simulink model "Primerpunto_a"  (R2017b)
settings: Solver=VariableStepAuto  StartTime=0.0  StopTime=80  RelTol=1e-3
settings Model: Creator=HP  LastModifiedBy=franj
settings CodeAppCC: StateflowObjectComments=on

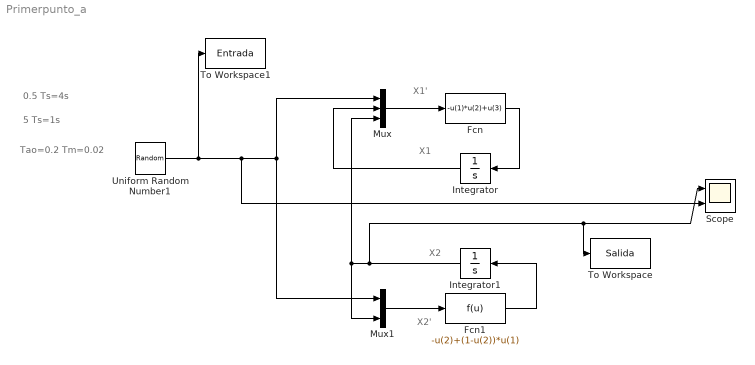
== system Primerpunto_a ==
  note: Tao=0.2
      | Tm=0.02
  note: 5 Ts=1s
  note: 0.5 Ts=4s
  note: X2'
  note: X2
  note: X1
  note: X1'
  Fcn : Fcn  Expr=-u(1)*u(2)+u(3)
  Fcn1 : Fcn  Expr=-u(2)+(1-u(2))*u(1)
  Integrator : Integrator
  Integrator1 : Integrator
  Mux : Mux  Inputs=3
  Mux1 : Mux  Inputs=2
  Scope : Scope  NumInputPorts=2
  To Workspace : ToWorkspace  VariableName=Salida  SampleTime=0.02
  To Workspace1 : ToWorkspace  VariableName=Entrada  SampleTime=0.02
  Uniform Random Number1 : UniformRandomNumber  Minimum=0  Maximum=5  SampleTime=4
  wires:
  Fcn/1 -> Integrator/1
  Fcn1/1 -> Integrator1/1
  Mux/1 -> Fcn/1
  Uniform Random Number1/1 -> To Workspace1/1, Scope/2, Mux/1, Mux1/1
  Integrator/1 -> Mux/2
  Integrator1/1 -> To Workspace/1, Scope/1, Mux1/2, Mux/3
  Mux1/1 -> Fcn1/1
